simulink subsystem "thermal_subsystem_model"  (R2023a)
settings: Solver=VariableStepAuto  StartTime=0.0  StopTime=10.0  RelTol=1e-3
values from neighbouring files (symbols this model uses):
  air_cp = 1004    [cathode_subsystem_parameters.m]    (also in thermal_subsystem_parameters.m)
  air_HC_min = 10    [cathode_subsystem_parameters.m]    (also in thermal_subsystem_parameters.m)
  air_HC_nom = 100    [cathode_subsystem_parameters.m]    (also in thermal_subsystem_parameters.m)
  air_rho = 1.2    [cathode_subsystem_parameters.m]    (also in thermal_subsystem_parameters.m)
  air_vel_nom = 1    [cathode_subsystem_parameters.m]    (also in thermal_subsystem_parameters.m)
  coolant_initial_pressure = 0.111325    [cathode_subsystem_parameters.m]    (also in thermal_subsystem_parameters.m)
  coolant_initial_temperature = 293.15    [cathode_subsystem_parameters.m]    (also in thermal_subsystem_parameters.m)
  coolant_tube_D = 0.05    [cathode_subsystem_parameters.m]    (also in thermal_subsystem_parameters.m)
  radiator_area_air = 0.10260000000000001    (= 0.1026)    [cathode_subsystem_parameters.m]    (also in thermal_subsystem_parameters.m)
  radiator_area_fins = 2.5436250000000005    (= 2.543625)    [cathode_subsystem_parameters.m]    (also in thermal_subsystem_parameters.m)
  radiator_area_primary = 0.44452500000000011    (= 0.444525)    [cathode_subsystem_parameters.m]    (also in thermal_subsystem_parameters.m = 2 * radiator_tube_length * radiator_width * (radiator_fin_ro)
  radiator_n_tubes = 20    [cathode_subsystem_parameters.m]    (also in thermal_subsystem_parameters.m)
  radiator_tube_height = 0.0015    [cathode_subsystem_parameters.m]    (also in thermal_subsystem_parameters.m)
  radiator_tube_length = 0.45    [cathode_subsystem_parameters.m]    (also in thermal_subsystem_parameters.m)
  radiator_width = 0.025    [cathode_subsystem_parameters.m]    (also in thermal_subsystem_parameters.m)
  tcp_time_constant = 2    [cathode_subsystem_parameters.m]    (also in thermal_subsystem_parameters.m)
  tcv_orifice_diameter = 0.045    [cathode_subsystem_parameters.m]    (also in thermal_subsystem_parameters.m)
  tcv_time_constant = 0.2    [cathode_subsystem_parameters.m]    (also in thermal_subsystem_parameters.m)
libraries: fl_lib x60, nesl_utility x46, SimscapeFluids_lib x8
(part 2 of 2)

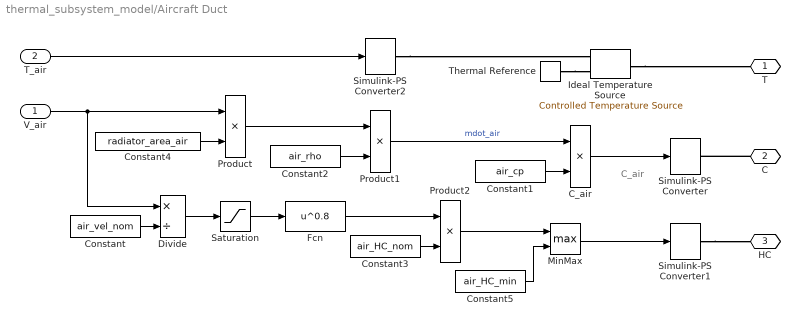
== system thermal_subsystem_model/Aircraft Duct ==
  note: C_air
  V_air : Inport
  T_air : Inport  Port=2
  C_air : Product
  Constant : Constant  Value=air_vel_nom
  Constant1 : Constant  Value=air_cp
  Constant2 : Constant  Value=air_rho
  Constant3 : Constant  Value=air_HC_nom
  Constant4 : Constant  Value=radiator_area_air
  Constant5 : Constant  Value=air_HC_min
  Divide : Product  Inputs=*/
  Fcn : Fcn  Expr=u^0.8
  Ideal Temperature Source : fl_lib/Thermal/Thermal Sources/Controlled Temperature Source
  MinMax : MinMax  Function=max  Inputs=2
  Product : Product
  Product1 : Product
  Product2 : Product
  Saturation : Saturate  UpperLimit=inf  LowerLimit=0
  Simulink-PS Converter : nesl_utility/Simulink-PS Converter  PhysicalDomain=network_engine_domain  SubClassName=ps_input  LeftPortType=input  RightPortType=output  PseudoPeriodic=off  Frequencies=[]  NoiseDistribution=none  NoiseParameters=[]  Unit=W/K  AffineConversion=off  FilteringAndDerivatives=zero  SimscapeFilterOrder=1  InputFilterTimeConstant=1  UdotUserProvided=1
  Simulink-PS Converter1 : nesl_utility/Simulink-PS Converter  PhysicalDomain=network_engine_domain  SubClassName=ps_input  LeftPortType=input  RightPortType=output  PseudoPeriodic=off  Frequencies=[]  NoiseDistribution=none  NoiseParameters=[]  Unit=W/(m^2*K)  AffineConversion=off  FilteringAndDerivatives=zero  SimscapeFilterOrder=1  InputFilterTimeConstant=1  UdotUserProvided=1
  Simulink-PS Converter2 : nesl_utility/Simulink-PS Converter  PhysicalDomain=network_engine_domain  SubClassName=ps_input  LeftPortType=input  RightPortType=output  PseudoPeriodic=off  Frequencies=[]  NoiseDistribution=none  NoiseParameters=[]  Unit=K  AffineConversion=on  FilteringAndDerivatives=zero  SimscapeFilterOrder=1  InputFilterTimeConstant=1  UdotUserProvided=1
  Thermal Reference : fl_lib/Thermal/Thermal Elements/Thermal Reference
  T : PMIOPort  Side=Right
  C : PMIOPort  Port=2  Side=Right
  HC : PMIOPort  Port=3  Side=Right
  wires:
  Saturation/1 -> Fcn/1
  Product1/1 -> C_air/1  "mdot_air"
  Constant4/1 -> Product/2
  Constant2/1 -> Product1/2
  Product/1 -> Product1/1
  C_air/1 -> Simulink-PS Converter/1
  Constant1/1 -> C_air/2
  T_air/1 -> Simulink-PS Converter2/1
  MinMax/1 -> Simulink-PS Converter1/1
  Constant5/1 -> MinMax/2
  Product2/1 -> MinMax/1
  Fcn/1 -> Product2/1
  Divide/1 -> Saturation/1
  Constant3/1 -> Product2/2
  Constant/1 -> Divide/2
  V_air/1 -> Divide/1, Product/1
  connections:
  Ideal Temperature Source/LConn1 -- T/RConn1
  Simulink-PS Converter2/RConn1 -- Ideal Temperature Source/RConn1
  Thermal Reference/LConn1 -- Ideal Temperature Source/RConn2
  Simulink-PS Converter1/RConn1 -- HC/RConn1
  C/RConn1 -- Simulink-PS Converter/RConn1

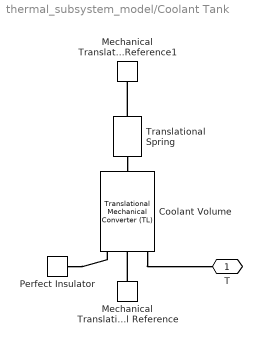
== system thermal_subsystem_model/Coolant Tank ==
  Coolant Volume : fl_lib/Thermal Liquid/Elements/Translational Mechanical Converter (TL)  mech_orientation=foundation.enum.MechOrientationTranslational.Positive  displacement_spec=foundation.enum.DisplacementSpec.Calculate  x0=x_init m  interface_area=A m^2  dead_volume=A * 0.001 m^3  environment_spec=foundation.enum.pressure_spec.specified  environment_pressure=coolant_initial_pressure MPa  dynamic_compressibility=simscape.enum.onoff.off  p0=env_p MPa  T0=coolant_initial_temperature K
      settings: InternalSimscapePortConfiguration="{\"Bottom\":[],\"Left\":[{\"id\":\"A\",\"label\":\"A\",\"type\":\"foundation.thermal_liquid.thermal_liquid\"},{\"id\":\"C\",\"label\":\"C\",\"type\":\"foundation.mechanical.translational.translational\"},{\"id\":\"H\",\"label\":\"H\",\"type\":\"foundation.thermal.thermal\"}],\"Right\":[{\"id\":\"R\",\"label\":\"R\",\"type\":\"foundation.mechanical.translational.translational\"}],\"Top\":[]}"
  Mechanical Translational Reference : fl_lib/Mechanical/Translational Elements/Mechanical Translational Reference
  Mechanical Translational Reference1 : fl_lib/Mechanical/Translational Elements/Mechanical Translational Reference
  Perfect Insulator : fl_lib/Thermal/Thermal Elements/Perfect Insulator  T_specify=off  T_priority=None  T=0 K  T_nominal_specify=off  T_nominal_unit=K  T_nominal_value=1
  Translational Spring : fl_lib/Mechanical/Translational Elements/Translational Spring  spr_rate=1e6 N/m  v_specify=off  v_priority=None  v=0 m/s  v_nominal_specify=off  v_nominal_unit=m/s  v_nominal_value=1  f_specify=off  f_priority=None  f=0 N  f_nominal_specify=off  f_nominal_unit=N  f_nominal_value=1  x_specify=off  x_priority=High  x=x_init m  x_nominal_specify=on  x_nominal_unit=m  x_nominal_value=x_init
  T : PMIOPort  Side=Right
  connections:
  Translational Spring/LConn1 -- Mechanical Translational Reference1/LConn1
  Translational Spring/RConn1 -- Coolant Volume/RConn1
  Perfect Insulator/LConn1 -- Coolant Volume/LConn3
  Mechanical Translational Reference/LConn1 -- Coolant Volume/LConn2
  Coolant Volume/LConn1 -- T/RConn1

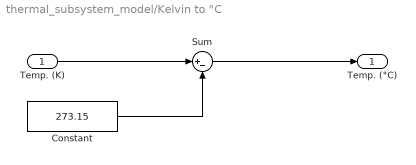
== system thermal_subsystem_model/Kelvin to °C ==
  Temp. (K) : Inport
  Constant : Constant  Value=273.15
  Sum : Sum  Inputs=|+-
  Temp. (°C) : Outport
  wires:
  Temp. (K)/1 -> Sum/1
  Sum/1 -> Temp. (°C)/1
  Constant/1 -> Sum/2

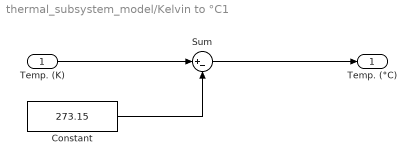
== system thermal_subsystem_model/Kelvin to °C1 ==
  Temp. (K) : Inport
  Constant : Constant  Value=273.15
  Sum : Sum  Inputs=|+-
  Temp. (°C) : Outport
  wires:
  Temp. (K)/1 -> Sum/1
  Sum/1 -> Temp. (°C)/1
  Constant/1 -> Sum/2

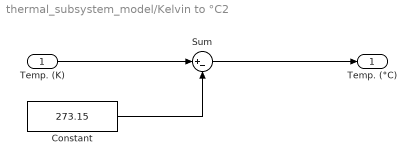
== system thermal_subsystem_model/Kelvin to °C2 ==
  Temp. (K) : Inport
  Constant : Constant  Value=273.15
  Sum : Sum  Inputs=|+-
  Temp. (°C) : Outport
  wires:
  Temp. (K)/1 -> Sum/1
  Sum/1 -> Temp. (°C)/1
  Constant/1 -> Sum/2

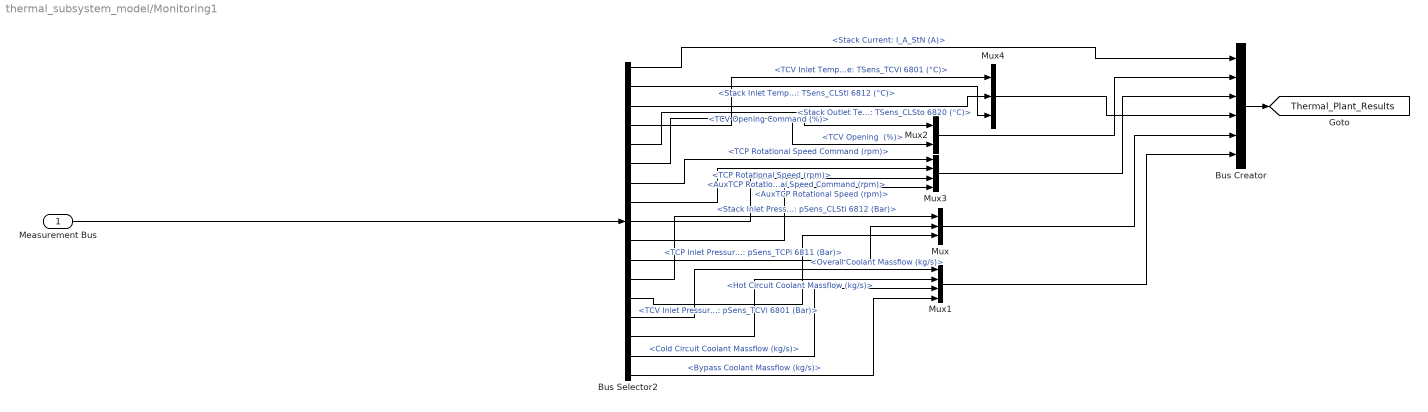
== system thermal_subsystem_model/Monitoring1 ==
  Measurement Bus : Inport
  Bus Creator : BusCreator  Inputs=6
  Bus Selector2 : BusSelector  OutputSignals="Stack Current: I_A_StN (A),Stack Inlet Temperature: TSens_CLSti 6812 (°C),Stack Outlet Temperature: TSens_CLSto 6820 (°C),TCV Inlet Temperature: TSens_TCVi 6801 (°C),TCV Opening Command (%),TCV Opening  (%),TCP Rotational Speed Command (rpm),TCP Rotational Speed (rpm),AuxTCP Rotational Speed Command (rpm),AuxTCP Rotational Speed (rpm),TCP Inlet Pressure: pSens_TCPi 6811 (Bar),Stack Inlet Pressure: pSens_CLSti 6812 (Bar),TCV Inlet Pressure: pSens_TCVi 6801 (Bar),Overall Coolant Massflow (kg/s),Hot Circuit Coolant Massflow (kg/s),Cold Circuit Coolant Massflow (kg/s),Bypass Coolant Massflow (kg/s)"
  Mux : Mux  Inputs=3
  Mux1 : Mux
  Mux2 : Mux  Inputs=2
  Mux3 : Mux
  Mux4 : Mux  Inputs=3
  tag scope: Thermal_Plant_Results=global
  wires:
  Bus Creator/1 -> [Thermal_Plant_Results]
  Bus Selector2/4 -> Mux4/1  "<TCV Inlet Temperature: TSens_TCVi 6801 (°C)>"
  Bus Selector2/1 -> Bus Creator/1  "<Stack Current: I_A_StN (A)>"
  Bus Selector2/12 -> Mux/1  "<Stack Inlet Pressure: pSens_CLSti 6812 (Bar)>"
  Bus Selector2/16 -> Mux1/3  "<Cold Circuit Coolant Massflow (kg/s)>"
  Bus Selector2/5 -> Mux2/1  "<TCV Opening Command (%)>"
  Bus Selector2/8 -> Mux3/2  "<TCP Rotational Speed (rpm)>"
  Bus Selector2/17 -> Mux1/4  "<Bypass Coolant Massflow (kg/s)>"
  Mux1/1 -> Bus Creator/6
  Bus Selector2/14 -> Mux1/1  "<Overall Coolant Massflow (kg/s)>"
  Bus Selector2/13 -> Mux/3  "<TCV Inlet Pressure: pSens_TCVi 6801 (Bar)>"
  Bus Selector2/15 -> Mux1/2  "<Hot Circuit Coolant Massflow (kg/s)>"
  Mux/1 -> Bus Creator/5
  Bus Selector2/6 -> Mux2/2  "<TCV Opening  (%)>"
  Bus Selector2/2 -> Mux4/3  "<Stack Inlet Temperature: TSens_CLSti 6812 (°C)>"
  Bus Selector2/9 -> Mux3/3  "<AuxTCP Rotational Speed Command (rpm)>"
  Measurement Bus/1 -> Bus Selector2/1
  Mux2/1 -> Bus Creator/2
  Bus Selector2/3 -> Mux4/2  "<Stack Outlet Temperature: TSens_CLSto 6820 (°C)>"
  Bus Selector2/7 -> Mux3/1  "<TCP Rotational Speed Command (rpm)>"
  Mux3/1 -> Bus Creator/3
  Bus Selector2/11 -> Mux/2  "<TCP Inlet Pressure: pSens_TCPi 6811 (Bar)>"
  Mux4/1 -> Bus Creator/4
  Bus Selector2/10 -> Mux3/4  "<AuxTCP Rotational Speed (rpm)>"

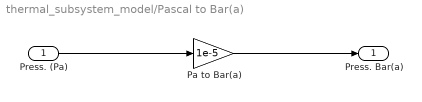
== system thermal_subsystem_model/Pascal to Bar(a) ==
  Press. (Pa) : Inport
  Pa to Bar(a) : Gain  Gain=1e-5
  Press. Bar(a) : Outport
  wires:
  Press. (Pa)/1 -> Pa to Bar(a)/1
  Pa to Bar(a)/1 -> Press. Bar(a)/1

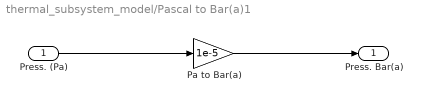
== system thermal_subsystem_model/Pascal to Bar(a)1 ==
  Press. (Pa) : Inport
  Pa to Bar(a) : Gain  Gain=1e-5
  Press. Bar(a) : Outport
  wires:
  Press. (Pa)/1 -> Pa to Bar(a)/1
  Pa to Bar(a)/1 -> Press. Bar(a)/1

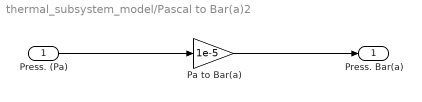
== system thermal_subsystem_model/Pascal to Bar(a)2 ==
  Press. (Pa) : Inport
  Pa to Bar(a) : Gain  Gain=1e-5
  Press. Bar(a) : Outport
  wires:
  Press. (Pa)/1 -> Pa to Bar(a)/1
  Pa to Bar(a)/1 -> Press. Bar(a)/1

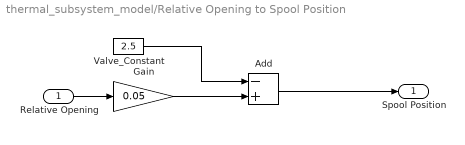
== system thermal_subsystem_model/Relative Opening to Spool Position ==
  Relative Opening : Inport
  Add : Sum  Inputs=-+
  Gain : Gain  Gain=0.05
  Valve_Constant : Constant  Value=2.5
  Spool Position : Outport
  wires:
  Add/1 -> Spool Position/1
  Valve_Constant/1 -> Add/1
  Relative Opening/1 -> Gain/1
  Gain/1 -> Add/2
